simulink model "Galvo_sys_v11_LessCallbacks"  (R2013a)
settings: Solver=ode45  StartTime=0.0  StopTime=SimEnd  MaxStep=1e-6  RelTol=1e-3
PreLoadFcn:
  | %$SimEnd = evalin('base','SimEnd');
  | %$Kp_cc = evalin('base',paramCtrl.Kp_cc);
  | %CC_EN = 1;
  | %Kp_ccMod = Kp_cc;
PostLoadFcn:
  | %scopes = find_system(gcs, 'BlockType', 'SignalViewerScope');
  | 
  | %for i=1:length(scopes)
  | %  set_param(scopes{i},'open','off');
  | %end
InitFcn:
  | %Kp_cc=evalin('base',paramCtrl.Kp_cc);
  | %Kp_ccMod = Kp_cc*CC_EN;
undefined symbols (not defined in the file or in its folder): Kp_ccMod
libraries: simulink x2
settings Model: BufferReuse=off  Creator=mainster  LastModifiedBy=mainster
settings OptimizationCC: InlineParams=on  BufferReuse=off
settings DebuggingCC: InitInArrayFormatMsg=none

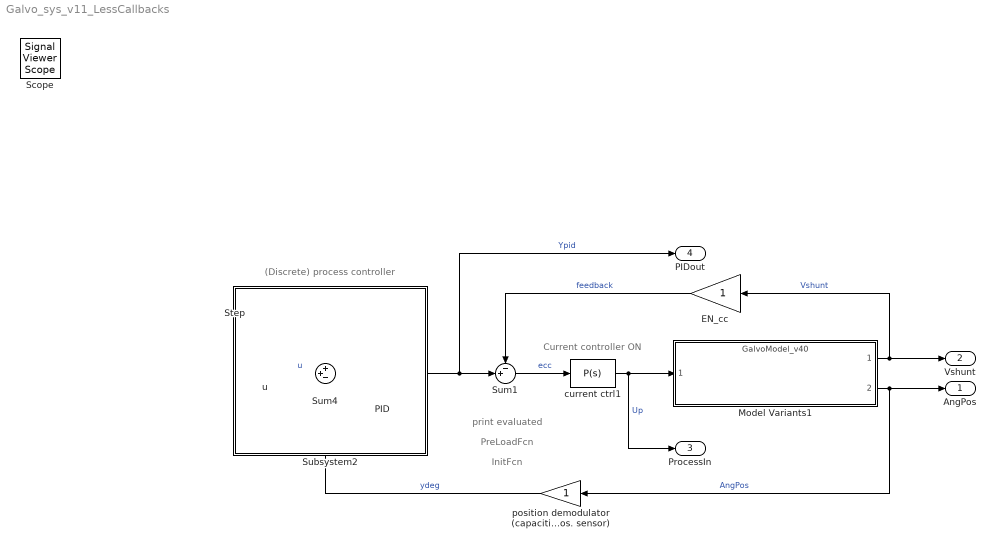
== system Galvo_sys_v11_LessCallbacks ==
  note: (Discrete) process controller
  note: Current controller ON
  note: print evaluated
  note: PreLoadFcn
  note: InitFcn
  u : Inport
  EN_cc : Gain
  Model Variants1 : ModelReference  ModelNameDialog=GalvoModel_v40.slx  SimulationMode=Normal  OverrideUsingVariant=Galvo_v40  ModelReferenceVersion=1.28  CopyOfModelName=GalvoModel_v40.slx  DefaultDataLogging=on
      mask init:
      | % 
      | % evalin('base', ['param=loadGalvoParam(' strrep(modVers(2:end-1),'.','') ');'])
      | % 
      | % switch modVers(1:2)
      | %     case 'v4'
      | %                 JR=evalin('base','param.JR');
      | %                 KMT=evalin('base','param.KMT');
      | %                 Rc=evalin('base','param.Rc');
      | %                 Lc=evalin('base','param.Lc');
      | %                 KFR=evalin('base','param.KFR');
      | %                 KTB=evalin('base','param.KTB');
      | %                 KBM=evalin('base','param.KBM');
      | %                 Rsh=evalin('base','param.Rsh');
      | %     case 'v3'
      | % 
      | %                 RIN=evalin('base','param.RIN');
      | %                 TRC=evalin('base','param.TRC');
      | %                 CR=evalin('base','param.CR');
      | %                 CL=evalin('base','param.CL');
      | %                 FR=evalin('base','param.FR');
      | %                 KTR=evalin('base','param.KTR');
      | %                 BEM=evalin('base','param.BEM');
      | %                 SHR=evalin('base','param.SHR');
      | %     otherwise
      | % 
      | % end
      | % 
      | % set_param(gcb, 'OverrideUsingVariant',sprintf('Galvo_%s',strrep(modVers,'.','')))
      | %
      settings: AttributesFormatString=%<ActiveVariant>
      mask Display:
      | str=sprintf('%s',get(gcbh,'ModelName'));
      | port_label('input', 1, 'VCoil','texmode','on')
      | color('blue');
      | port_label('output', 1, 'VShunt','texmode','on')
      | color('black');
      | port_label('output', 2, 'AngPos')
      | %text(.05,.98,['{\fontsize{12}\it\bf' strrep(str,'_',' ') '}'],'horizontalAlignment','left','verticalAlignment','top','texmode','on')
      | text(.015,.98,['{\fontsize{12}\it\bf' strrep(str,'_','\_') '}'],'horizontalAlignment','left','verticalAlignment','top','texmode','on')
  PID : simulink/Continuous/PID Controller  Controller=PID  TimeDomain=Continuous-time  SampleTime=1  IntegratorMethod=Forward Euler  FilterMethod=Forward Euler  Form=Ideal  P=1.27962052694162  I=26.6543981133797  D=0.00484773093084055  N=19608.9145050565  InitialConditionSource=internal  InitialConditionForIntegrator=0  InitialConditionForFilter=0  ExternalReset=none  IgnoreLimit=on  LimitOutput=on  UpperSaturationLimit=2.5  LowerSaturationLimit=-2.5  LinearizeAsGain=on  AntiWindupMode=back-calculation  Kb=0.8  TrackingMode=off  Kt=0  PParamMin=[]  PParamMax=[]  IParamMin=[]  IParamMax=[]  DParamMin=[]  DParamMax=[]  NParamMin=[]  NParamMax=[]  KbParamMin=[]  KbParamMax=[]  KtParamMin=[]  KtParamMax=[]  POutMin=[]  POutMax=[]  IOutMin=[]  IOutMax=[]  DOutMin=[]  DOutMax=[]  NOutMin=[]  NOutMax=[]  KbOutMin=[]  KbOutMax=[]  KtOutMin=[]  KtOutMax=[]  IntegratorOutMin=[]  IntegratorOutMax=[]  FilterOutMin=[]  FilterOutMax=[]  SumOutMin=[]  SumOutMax=[]  SumI1OutMin=[]  SumI1OutMax=[]  SumI2OutMin=[]  SumI2OutMax=[]  SumI3OutMin=[]  SumI3OutMax=[]  SumDOutMin=[]  SumDOutMax=[]  SaturationOutMin=[]  SaturationOutMax=[]  IntegratorContinuousStateAttributes=''  IntegratorStateMustResolveToSignalObject=off  IntegratorRTWStateStorageClass=Auto  FilterContinuousStateAttributes=''  FilterStateMustResolveToSignalObject=off  FilterRTWStateStorageClass=Auto
  Step : Step  Time=1e-3  SampleTime=0  ZeroCross=off
      settings: AttributesFormatString=Ampl.: %<After>
  Subsystem2 : Subsystem  mask{d=0}
      mask Display: disp('')
  Sum1 : Sum  Inputs=-+|
  Sum4 : Sum  Inputs=++-
  current ctrl1 : simulink/Continuous/PID Controller  Controller=P  TimeDomain=Continuous-time  SampleTime=1  IntegratorMethod=Forward Euler  FilterMethod=Forward Euler  Form=Parallel  P=Kp_ccMod  I=0.7525  D=0.156  N=100  InitialConditionSource=internal  InitialConditionForIntegrator=0  InitialConditionForFilter=0  ExternalReset=none  LimitOutput=on  UpperSaturationLimit=25  LowerSaturationLimit=-25  LinearizeAsGain=on  AntiWindupMode=none  Kb=1  TrackingMode=off  Kt=1  PParamMin=[]  PParamMax=[]  IParamMin=[]  IParamMax=[]  DParamMin=[]  DParamMax=[]  NParamMin=[]  NParamMax=[]  KbParamMin=[]  KbParamMax=[]  KtParamMin=[]  KtParamMax=[]  POutMin=[]  POutMax=[]  IOutMin=[]  IOutMax=[]  DOutMin=[]  DOutMax=[]  NOutMin=[]  NOutMax=[]  KbOutMin=[]  KbOutMax=[]  KtOutMin=[]  KtOutMax=[]  IntegratorOutMin=[]  IntegratorOutMax=[]  FilterOutMin=[]  FilterOutMax=[]  SumOutMin=[]  SumOutMax=[]  SumI1OutMin=[]  SumI1OutMax=[]  SumI2OutMin=[]  SumI2OutMax=[]  SumI3OutMin=[]  SumI3OutMax=[]  SumDOutMin=[]  SumDOutMax=[]  SaturationOutMin=[]  SaturationOutMax=[]  IntegratorContinuousStateAttributes=''  IntegratorStateMustResolveToSignalObject=off  IntegratorRTWStateStorageClass=Auto  FilterContinuousStateAttributes=''  FilterStateMustResolveToSignalObject=off  FilterRTWStateStorageClass=Auto
  position demodulator (capacitive angular pos. sensor) : Gain
  AngPos : Outport
  Vshunt : Outport  Port=2
  ProcessIn : Outport  Port=3
  PIDout : Outport  Port=4
  Scope : SignalViewerScope  IOType=viewer  NumInputPorts=4  LegendLocations=|  RefreshTime=0.035000
      | 0.83092     0.92738     0.13817    0.024722
      | 0.86756     0.69252     0.10153    0.024722
      | 0.84924      0.4589     0.11985    0.024722
      | 0.81412     0.22404     0.13817    0.024722
      settings: ShowLegends=on  TimeRange=0.03  YMin=-0.5~-10~-1~-0.5  YMax=1.5~30~3~1  MaxDataPoints=75000
  wires:
  Sum4/1 -> PID/1
  Step/1 -> Sum4/1
  u/1 -> Sum4/2  "u"
  position demodulator (capacitive angular pos. sensor)/1 -> Sum4/3  "ydeg"
  Sum1/1 -> current ctrl1/1  "ecc"
  Model Variants1/1 -> Vshunt/1, EN_cc/1  "Vshunt"
  current ctrl1/1 -> ProcessIn/1, Model Variants1/1  "Up"
  PID/1 -> PIDout/1, Sum1/2  "Ypid"
  Model Variants1/2 -> AngPos/1, position demodulator (capacitive angular pos. sensor)/1  "AngPos"
  EN_cc/1 -> Sum1/1  "feedback"

== system Galvo_sys_v11_LessCallbacks/Subsystem2 ==
